simulink model "ee407_hw2_q3f"  (R2020a)
settings: Solver=FixedStepAuto  StartTime=0.0  StopTime=20  FixedStep=1e-5  RelTol=1e-3
undefined symbols (not defined in the file): n1, n2, y1
settings Model: Creator=iky  LastModifiedBy=iky

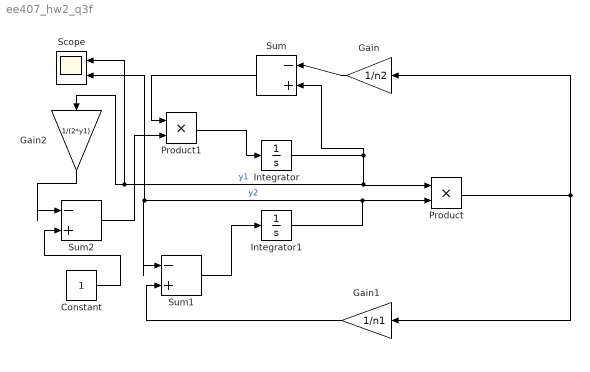
== system ee407_hw2_q3f ==
  Constant : Constant
  Gain : Gain  Gain=1/n2
  Gain1 : Gain  Gain=1/n1
  Gain2 : Gain  Gain=1/(2*y1)
  Integrator : Integrator  InitialCondition=400
  Integrator1 : Integrator  InitialCondition=100
  Product : Product
  Product1 : Product
  Scope : Scope  NumInputPorts=2
  Sum : Sum  Inputs=|-+
  Sum1 : Sum  Inputs=|-+
  Sum2 : Sum  Inputs=|-+
  wires:
  Integrator1/1 -> Product/2, Scope/2, Sum1/1  "y2"
  Integrator/1 -> Scope/1, Gain2/1, Product/1, Sum/2  "y1"
  Product/1 -> Gain/1, Gain1/1
  Gain/1 -> Sum/1
  Sum/1 -> Product1/1
  Constant/1 -> Sum2/2
  Sum2/1 -> Product1/2
  Product1/1 -> Integrator/1
  Sum1/1 -> Integrator1/1
  Gain1/1 -> Sum1/2
  Gain2/1 -> Sum2/1
